simulink model "Solar_power_system_for_home"  (R2023a)
settings: Solver=VariableStepAuto  StartTime=0.0  StopTime=5.0  RelTol=1e-3
libraries: spsSeriesRLCBranchLib x6, spsVoltageMeasurementLib x3, spsDiodeLib x1, spsIGBTDiodeLib x1, spsPVArrayLib x1, spsPWMGenerator2LevelLib x1, spsUniversalBridgeLib x1, sps_lib x1
settings Model: Creator=HIRUSHA GIMHAN  LastModifiedBy=HIRUSHA GIMHAN

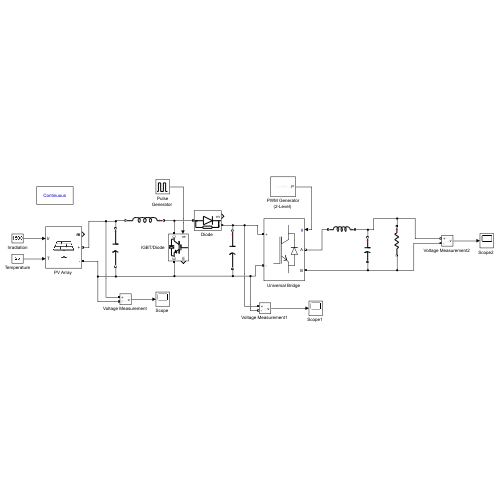
[thumbnail: Simulink's stored preview of the top-level diagram]
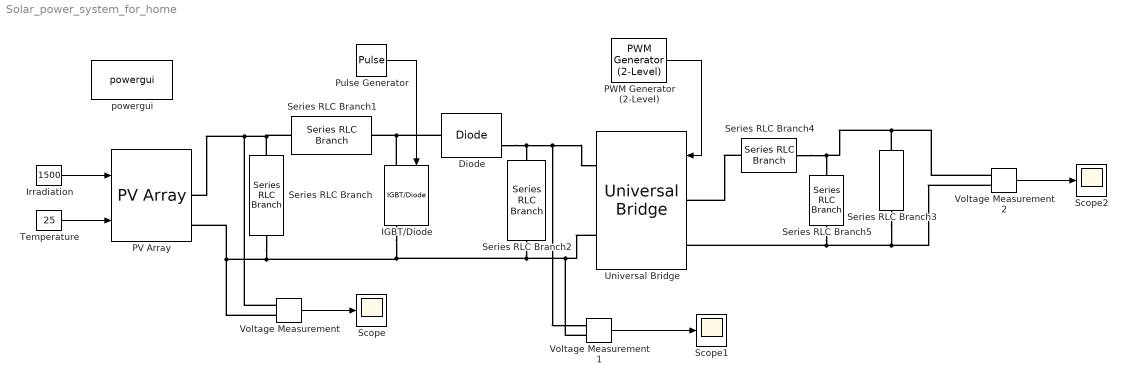
== system Solar_power_system_for_home ==
  "Diode " : spsDiodeLib/Diode  Ron=0.001  Lon=0  Vf=0.8  IC=0  UseSnubber=0  Rs=500  Cs=250e-8  Measurements=on
  "IGBT/Diode " : spsIGBTDiodeLib/IGBT//Diode  Ron=1e-3  Rs=1e4  Cs=inf  Measurements=on
  Irradiation : Constant  Value=1500
  "PV Array " : spsPVArrayLib/PV Array  Npar=20  Nser=5  PlotType=array @ 1000 W/m2 & specified temperatures  S_vec="[ 1000  500  100 ]"  Temp_C_vec="[ 45 25  ]"  ModuleName=American Solar Wholesale ASW-250P  PlotWhenSelected=off  Pm=249.92  Ncell=72  Voc=43.22  Isc=7.76  Vm=35.2  Im=7.1  beta_Voc_pc=-0.30278  alpha_Isc_pc=0.035271  beta_Voc=-0.13086  alpha_Isc=0.002737  IL=7.7892  I0=2.8627e-11  nI=0.8891  Rsh=111.8733  Rs=0.42123  RobustModel=off  RobustCellTemperature=313.3991  BAL=on  Tc=1e-10  Tfilter=5e-5
  "PWM Generator (2-Level) " : spsPWMGenerator2LevelLib/PWM Generator (2-Level)  ModulatorType=Single-phase full-bridge (4 pulses)  ModulatorMode=Unsynchronized  Fc=27*60  Pc=90  nF=27  MinMax="[ -1  1 ]"  SamplingTechnique=Natural  ModulatingSignals=on  m=0.8  Freq=51  Phase=0  Ts=0  ShowCarrierOutport=off
  "Pulse Generator " : DiscretePulseGenerator  PulseType=Time based  Period=1/1500  PulseWidth=61.8
  "Scope " : Scope
  "Scope1 " : Scope
  "Scope2 " : Scope
  Series RLC Branch : spsSeriesRLCBranchLib/Series RLC Branch  LConnTagsString=__new0  RConnTagsString=__new0  BranchType=C  Resistance=1  Inductance=1e-3  SetiL0=off  InitialCurrent=0  Capacitance=2.2e-3  Setx0=off  InitialVoltage=0  Measurements=None
  Series RLC Branch1 : spsSeriesRLCBranchLib/Series RLC Branch  LConnTagsString=__new0  RConnTagsString=__new0  BranchType=L  Resistance=1  Inductance=0.02  SetiL0=off  InitialCurrent=0  Capacitance=0.006  Setx0=off  InitialVoltage=0  Measurements=None
  Series RLC Branch2 : spsSeriesRLCBranchLib/Series RLC Branch  LConnTagsString=__new0  RConnTagsString=__new0  BranchType=C  Resistance=1  Inductance=1e-3  SetiL0=off  InitialCurrent=0  Capacitance=0.47  Setx0=off  InitialVoltage=0  Measurements=None
  Series RLC Branch3 : spsSeriesRLCBranchLib/Series RLC Branch  LConnTagsString=__new0  RConnTagsString=__new0  BranchType=R  Resistance=4  Inductance=1e-3  SetiL0=off  InitialCurrent=0  Capacitance=0.006  Setx0=off  InitialVoltage=0  Measurements=None
  Series RLC Branch4 : spsSeriesRLCBranchLib/Series RLC Branch  LConnTagsString=__new0  RConnTagsString=__new0  BranchType=L  Resistance=0.06  Inductance=0.002  SetiL0=off  InitialCurrent=0  Capacitance=0.006  Setx0=off  InitialVoltage=0  Measurements=None
  Series RLC Branch5 : spsSeriesRLCBranchLib/Series RLC Branch  LConnTagsString=__new0  RConnTagsString=__new0  BranchType=C  Resistance=1  Inductance=1e-3  SetiL0=off  InitialCurrent=0  Capacitance=0.006  Setx0=off  InitialVoltage=0  Measurements=None
  Temperature : Constant  Value=25
  "Universal Bridge " : spsUniversalBridgeLib/Universal Bridge  Arms=2  SnubberResistance=1e5  SnubberCapacitance=inf  Device=IGBT / Diodes  Ron=1e-3  Lon=0  ForwardVoltages="[  0  0  ]"  ForwardVoltage=0  GTOparameters=[ 10e-6 , 20e-6 ]  IGBTparameters=[ 1e-6 , 2e-6 ]  Measurements=None  Measurements_2=None  converterType=Rectifier
  "Voltage Measurement " : spsVoltageMeasurementLib/Voltage Measurement  PhasorSimulation=off  OutputType=Complex  PSBequivalent=0
  "Voltage Measurement1 " : spsVoltageMeasurementLib/Voltage Measurement  PhasorSimulation=off  OutputType=Complex  PSBequivalent=0
  "Voltage Measurement2 " : spsVoltageMeasurementLib/Voltage Measurement  PhasorSimulation=off  OutputType=Complex  PSBequivalent=0
  powergui : sps_lib/powergui  Priority=1  SimulationMode=Continuous  SampleTime=50e-6  frequency=60  Iterations=50  frequencyindice=0  Pbase=100e6  ErrMax=1e-4  UnitsV=kV  UnitsW=MW  buscounter=0  FunctionMessages=off  echomessages=off  EnableUseOfTLC=off  CurrentSourceSwitches=off  DisableSnubberDevices=off  DisableRonSwitches=off  DisableVfSwitches=off  DisplayEquations=off  AutomaticDiscreteSolvers=off  SolverType=Tustin/Backward Euler (TBE)  Interpol=off  ExternalGateDelay=off  methode=off  Ts=100  x0status=blocks  SPID=on  SwTol=0  HookPort=off  NonlinearTolerance=1e-4  nMaxIteration=100  ContinueOnMaxIteration=off  RestoreLinks=warning  ResistiveCurrentMeasurement=off  Frange=[0:2:500]  Ylog=off  Xlog=on  ShowGrid=off  save=off  variable=ZData  structure=0  ZoomFFT=off  StartTime=0.0  cycles=1  DisplayStyle=1  fundamental=60  FreqAxis=off  MaxFrequency=1000  frequencyindicesteady=1  RmsSteady=1  display=off
  wires:
  Temperature/1 -> "PV Array "/2
  Irradiation/1 -> "PV Array "/1
  "Voltage Measurement "/1 -> "Scope "/1
  "PWM Generator (2-Level) "/1 -> "Universal Bridge "/1
  "Voltage Measurement1 "/1 -> "Scope1 "/1
  "Pulse Generator "/1 -> "IGBT/Diode "/1
  "Voltage Measurement2 "/1 -> "Scope2 "/1
  connections:
  Series RLC Branch/LConn1 -- Series RLC Branch1/RConn1 -- "Voltage Measurement "/LConn1 -- "PV Array "/RConn1
  "Voltage Measurement "/LConn2 -- "Voltage Measurement1 "/LConn2 -- "Universal Bridge "/RConn2 -- Series RLC Branch2/RConn1 -- "IGBT/Diode "/RConn1 -- Series RLC Branch/RConn1 -- "PV Array "/RConn2
  "Diode "/LConn1 -- "IGBT/Diode "/LConn1 -- Series RLC Branch1/LConn1
  "Diode "/RConn1 -- "Voltage Measurement1 "/LConn1 -- "Universal Bridge "/RConn1 -- Series RLC Branch2/LConn1
  Series RLC Branch4/RConn1 -- "Universal Bridge "/LConn1
  Series RLC Branch4/LConn1 -- "Voltage Measurement2 "/LConn1 -- Series RLC Branch3/LConn1 -- Series RLC Branch5/LConn1
  Series RLC Branch5/RConn1 -- "Voltage Measurement2 "/LConn2 -- Series RLC Branch3/RConn1 -- "Universal Bridge "/LConn2
